simulink model "nullspace_kinctrlkinova"  (R2021a)
settings: Solver=VariableStepAuto  StartTime=0.0  StopTime=30  RelTol=1e-3
values from neighbouring files (symbols this model uses):
  k2 = 1    [nullspace_script.m]    (also in sim_q2.m)
  k3 = 1    [nullspace_script.m]    (also in sim_q2.m)
  q0 = [0, 15, 180, -130, 0, 55, 90]    [mdl_kinovagen3_trab2.m]    (also in mdl_planar_2r.m = [-pi/20, -pi/2])
libraries: roblocks x6
settings Model: Creator=Guga  LastModifiedBy=Guga

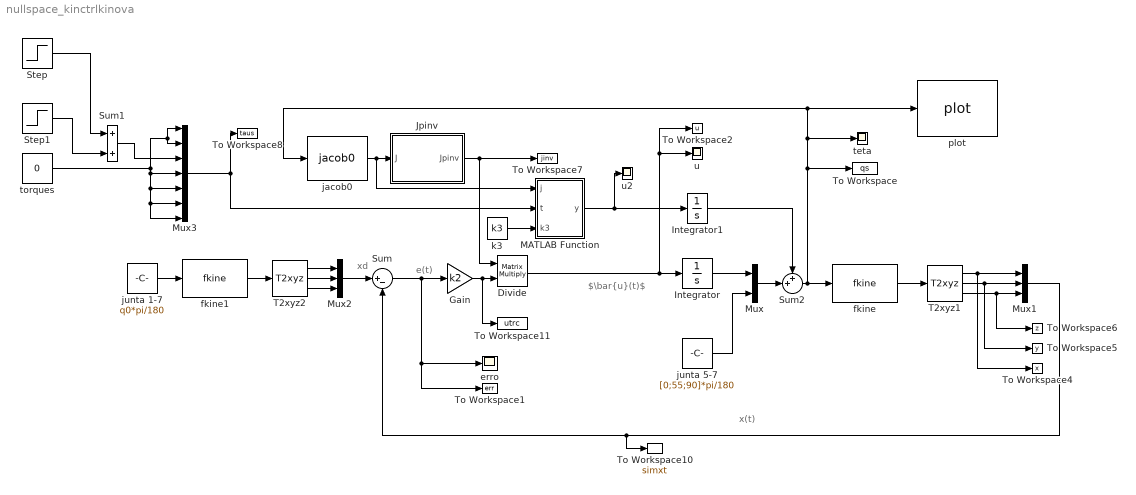
== system nullspace_kinctrlkinova ==
  note: x(t)
  note: xd
  note: e(t)
  note: $\bar{u}(t)$
  Divide : Product  Inputs=**  Multiplication=Matrix(*)
  Gain : Gain  Gain=k2
  Integrator : Integrator  InitialCondition=q0(1:4)*pi/180
  Integrator1 : Integrator  InitialCondition=[0,0,0,0,0,0,0]
  Jpinv : MATLAB Function  TreatAsAtomicUnit=on
  MATLAB Function : MATLAB Function  TreatAsAtomicUnit=on
  Mux : Mux  Inputs=2
  Mux1 : Mux  Inputs=3
  Mux2 : Mux  Inputs=3
  Mux3 : Mux  Inputs=7
  Step : Step  Time=2  SampleTime=0
  Step1 : Step  Time=3  After=-1  SampleTime=0
  Sum : Sum  Inputs=|+-
  Sum1 : Sum
  Sum2 : Sum  Inputs=++|
  T2xyz1 : roblocks/Toolbox/T2xyz
  T2xyz2 : roblocks/Toolbox/T2xyz
  To Workspace : ToWorkspace  VariableName=qs  SaveFormat=Timeseries  SampleTime=-1
  To Workspace1 : ToWorkspace  VariableName=err  SaveFormat=Timeseries  SampleTime=-1
  To Workspace10 : ToWorkspace  VariableName=simxt  SaveFormat=Timeseries  SampleTime=-1
  To Workspace11 : ToWorkspace  VariableName=utrc  SaveFormat=Timeseries  SampleTime=-1
  To Workspace2 : ToWorkspace  VariableName=u  SaveFormat=Timeseries  SampleTime=-1
  To Workspace4 : ToWorkspace  VariableName=x  SaveFormat=Timeseries  SampleTime=-1
  To Workspace5 : ToWorkspace  VariableName=y  SaveFormat=Timeseries  SampleTime=-1
  To Workspace6 : ToWorkspace  VariableName=z  SaveFormat=Timeseries  SampleTime=-1
  To Workspace7 : ToWorkspace  VariableName=jinv  SaveFormat=Timeseries  SampleTime=-1
  To Workspace8 : ToWorkspace  VariableName=taus  SaveFormat=Timeseries  SampleTime=-1
  erro : Scope
  fkine : roblocks/Arm/fkine  robot=gen3
  fkine1 : roblocks/Arm/fkine  robot=gen3
  "jacob0 " : roblocks/Arm/jacob0   robot=gen3
  junta 1-7 : Constant  Value=q0*pi/180
  junta 5-7 : Constant  Value=[0;55;90]*pi/180
  k3 : Constant  Value=k3
  plot : roblocks/Arm/plot  robot=gen3  fps=5  holdplot=on
  teta : Scope
  torques : Constant  Value=0
  u : Scope
  u2 : Scope
  wires:
  "jacob0 "/1 -> MATLAB Function/1(j), Jpinv/1(J)
  Gain/1 -> To Workspace11/1, Divide/2
  Integrator/1 -> Mux/1
  Sum/1 -> Gain/1, erro/1, To Workspace1/1
  Divide/1 -> To Workspace2/1, u/1, Integrator/1
  Jpinv/1(Jpinv) -> To Workspace7/1, Divide/1
  Sum2/1 -> To Workspace/1, teta/1, plot/1, "jacob0 "/1, fkine/1
  junta 5-7/1 -> Mux/2
  T2xyz1/3 -> To Workspace6/1, Mux1/3
  T2xyz1/2 -> To Workspace5/1, Mux1/2
  T2xyz1/1 -> Mux1/1, To Workspace4/1
  fkine/1 -> T2xyz1/1
  Mux1/1 -> To Workspace10/1, Sum/2
  junta 1-7/1 -> fkine1/1
  fkine1/1 -> T2xyz2/1
  Mux2/1 -> Sum/1
  T2xyz2/1 -> Mux2/1
  T2xyz2/2 -> Mux2/2
  T2xyz2/3 -> Mux2/3
  Mux3/1 -> To Workspace8/1, MATLAB Function/2(t)
  torques/1 -> Mux3/5, Mux3/6, Mux3/7, Mux3/4, Mux3/2, Mux3/1
  Sum1/1 -> Mux3/3
  Step/1 -> Sum1/1
  Step1/1 -> Sum1/2
  MATLAB Function/1(y) -> u2/1, Integrator1/1
  Integrator1/1 -> Sum2/1
  Mux/1 -> Sum2/2
  k3/1 -> MATLAB Function/3(k3)

== matlab function nullspace_kinctrlkinova/Jpinv ==
  data: J input; Jpinv output
function Jpinv = fcn(J)
%#codegen

Jpinv = pinv(J(1:3,1:4));

== matlab function nullspace_kinctrlkinova/MATLAB Function ==
  data: j input; y output; t input; k3 input
function y = fcn(j,t,k3)
    u = t.*(-2*k3);
    ji = pinv(j);
    y = (eye(7,7) - (ji*j))*u;
end
